simulink model "sysmod1"  (R2019a)
settings: Solver=ode23t  StartTime=0.0  StopTime=2  MaxStep=1e-6  MinStep=1e-7  RelTol=1e-3  EnableMultiTasking=on
values from neighbouring files (symbols this model uses):
  AedivR = pi*hp    (= 0.141371669412)    [setpara1.m]
  Dign = 1    [setpara1.m]
  Dm = 19    [setpara1.m]
  E_const = volpersec / E_spark    (= 5.35724220928e-09)    [setpara1.m]
  init_ediff = 50e-6    (= 5e-05)    [setpara1.m]
  Iref = 5    [setpara1.m]
  mm_dis = 100e-6    (= 0.0001)    [setpara1.m]
  Rsp = 1    [setpara1.m]
  SV = 35    [setpara1.m]
  SVoffset = 2    [setpara1.m]
  Td = Tign + Tm    (= 0.0002)    [setpara1.m]
  Tign = Dign / 100 * Tmach    (= 1e-05)    [setpara1.m]
  Tmach = 1/fmach    (= 0.001)    [setpara1.m]
  Vref = 70    [setpara1.m]
  w1 = 2*pi*f1    (= 62.8318530718)    [setpara1.m]
  wireRad = 90e-6    (= 9e-05)    [setpara1.m]
  wo = 2*pi*fo    (= 62.8318530718)    [setpara1.m]
libraries: powerlib x11, simulink x4
settings Model: Creator=FC Lab  LastModifiedBy=Prakhar
settings SolverCC: AlgebraicLoopSolver=LineSearch
settings DataIOCC: LimitDataPoints=on  ReturnWorkspaceOutputs=off
settings OptimizationCC: LifeSpan=inf
settings DebuggingCC: AllowSymbolicDim=off  SFUnexpectedBacktrackingDiag=warning  SFNoUnconditionalDefaultTransitionDiag=warning  SFExecutionAtInitializationDiag=none  ArithmeticOperatorsInVariantConditions=warning
settings ModelReferenceCC: PropagateSignalLabelsOutOfModel=off
settings SFSimCC: SimUseLocalCustomCode=off
settings RTWCC: RTWUseLocalCustomCode=off
settings CodeAppCC: StateflowObjectComments=on
settings GRTTargetCC: TargetLangStandard=C89/C90 (ANSI)
settings ConfigComp: CovMetricSettings=dw  CovHtmlReporting=on  CovSaveCumulativeToWorkspaceVar=on  CovSaveSingleToWorkspaceVar=on  CovExternalEMLEnable=off
settings SimscapeCC: SimscapeNormalizeSystem=off

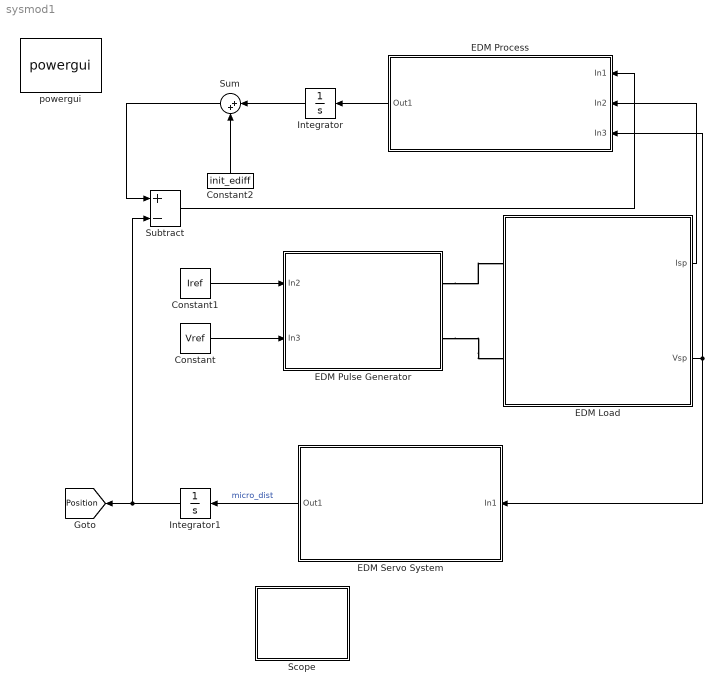
== system sysmod1 ==
  Constant : Constant  Value=Vref
  Constant1 : Constant  Value=Iref
  Constant2 : Constant  Value=init_ediff
  "EDM Load " : Subsystem
  EDM Process : Subsystem
  "EDM Pulse Generator " : Subsystem
  EDM Servo System : Subsystem
  Integrator : Integrator
  Integrator1 : Integrator
  "Scope " : Subsystem
  Subtract : Sum  Inputs=+-
  Sum : Sum  Inputs=|++
  powergui : powerlib/powergui  Priority=1  SimulationMode=Continuous  SampleTime=5e-07  frequency=60  Iterations=50  frequencyindice=0  Pbase=100e6  ErrMax=1e-4  UnitsV=kV  UnitsW=MW  buscounter=0  FunctionMessages=off  echomessages=off  EnableUseOfTLC=off  CurrentSourceSwitches=off  DisableSnubberDevices=off  DisableRonSwitches=off  DisableVfSwitches=off  DisplayEquations=off  AutomaticDiscreteSolvers=off  SolverType=Backward Euler  Interpol=off  ExternalGateDelay=off  methode=off  Ts=0  x0status=zero  SPID=on  SwTol=0  HookPort=off  NonlinearTolerance=0  nMaxIteration=15  ContinueOnMaxIteration=off  RestoreLinks=warning  ResistiveCurrentMeasurement=off  Frange=[0:2:500]  Ylog=off  Xlog=on  ShowGrid=off  save=off  variable=ZData  structure=ScopeData  ZoomFFT=off  StartTime=0.0  cycles=5  DisplayStyle=2  fundamental=50  FreqAxis=off  MaxFrequency=50000  frequencyindicesteady=1  RmsSteady=1  display=off
      settings: SourceProductName=Simscape Electrical
  tag scope: Position=global
  wires:
  Constant1/1 -> "EDM Pulse Generator "/1(In2)
  Constant/1 -> "EDM Pulse Generator "/2(In3)
  "EDM Load "/2(Vsp) -> EDM Servo System/1(In1), EDM Process/3(In3)
  EDM Process/1(Out1) -> Integrator/1
  EDM Servo System/1(Out1) -> Integrator1/1  "micro_dist"
  Integrator1/1 -> Subtract/2, [Position]
  Constant2/1 -> Sum/2
  Integrator/1 -> Sum/1
  Sum/1 -> Subtract/1
  Subtract/1 -> EDM Process/1(In1)
  "EDM Load "/1(Isp) -> EDM Process/2(In2)
  connections:
  "EDM Pulse Generator "/RConn1 -- "EDM Load "/LConn1
  "EDM Pulse Generator "/RConn2 -- "EDM Load "/LConn2

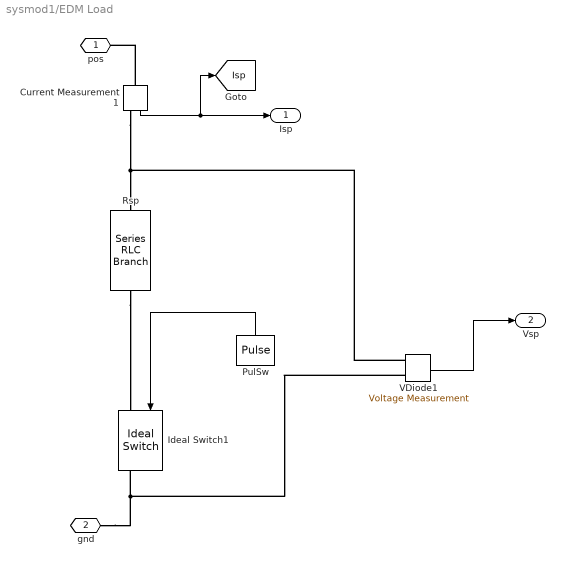
== system sysmod1/EDM Load  ==
  Current Measurement1 : powerlib/Measurements/Current Measurement  PhasorSimulation=off  OutputType=Complex  PSBequivalent=0
      settings: SourceProductName=Simscape Electrical
  Ideal Switch1 : powerlib/Power Electronics/Ideal Switch  Ron=0.001  Lon=0  IC=0  Rs=1e5  Cs=inf  Measurements=on
      settings: SourceProductName=Simscape Electrical
  PulSw : DiscretePulseGenerator  PulseType=Time based  Period=Tmach  PulseWidth=Dm  PhaseDelay=Tign
  Rsp : powerlib/Elements/Series RLC Branch  LConnTagsString=__new0  RConnTagsString=__new0  BranchType=R  Resistance=Rsp  Inductance=3e-6  SetiL0=off  InitialCurrent=0  Capacitance=1e-6  Setx0=off  InitialVoltage=0  Measurements=None
      settings: SourceProductName=Simscape Electrical
  VDiode1 : powerlib/Measurements/Voltage Measurement  PhasorSimulation=off  OutputType=Complex  PSBequivalent=0
      settings: SourceProductName=Simscape Electrical
  pos : PMIOPort  Side=Left
  gnd : PMIOPort  Port=2  Side=Left
  Isp : Outport
  Vsp : Outport  Port=2
  tag scope: Isp=global
  wires:
  PulSw/1 -> Ideal Switch1/1
  Current Measurement1/1 -> [Isp], Isp/1
  VDiode1/1 -> Vsp/1
  connections:
  gnd/RConn1 -- VDiode1/LConn2 -- Ideal Switch1/RConn1
  Current Measurement1/LConn1 -- pos/RConn1
  Current Measurement1/RConn1 -- VDiode1/LConn1 -- Rsp/LConn1
  Rsp/RConn1 -- Ideal Switch1/LConn1

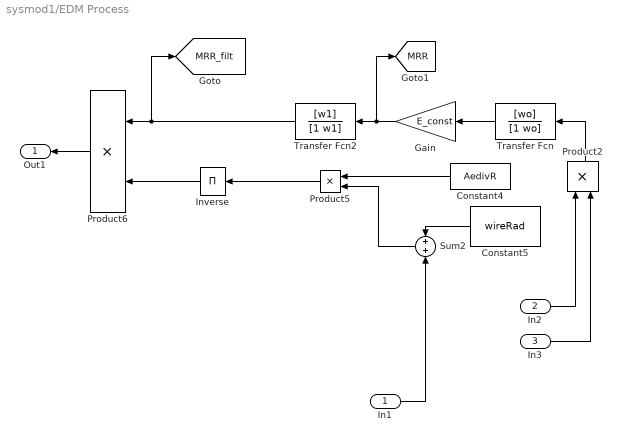
== system sysmod1/EDM Process ==
  In1 : Inport
  In2 : Inport  Port=2
  In3 : Inport  Port=3
  Constant4 : Constant  Value=AedivR
  Constant5 : Constant  Value=wireRad
  Gain : Gain  Gain=E_const
  "Inverse " : Product  Inputs=1
  Product2 : Product
  Product5 : Product
  Product6 : Product
  Sum2 : Sum
  Transfer Fcn : TransferFcn  Numerator=[wo]  Denominator=[1 wo]
  Transfer Fcn2 : TransferFcn  Numerator=[w1]  Denominator=[1 w1]
  Out1 : Outport
  tag scope: MRR=global, MRR_filt=global
  wires:
  Sum2/1 -> Product5/2
  Product6/1 -> Out1/1
  Constant4/1 -> Product5/1
  Product2/1 -> Transfer Fcn/1
  Constant5/1 -> Sum2/1
  "Inverse "/1 -> Product6/2
  Transfer Fcn/1 -> Gain/1
  Product5/1 -> "Inverse "/1
  Transfer Fcn2/1 -> [MRR_filt], Product6/1
  Gain/1 -> [MRR], Transfer Fcn2/1
  In1/1 -> Sum2/2
  In2/1 -> Product2/1
  In3/1 -> Product2/2

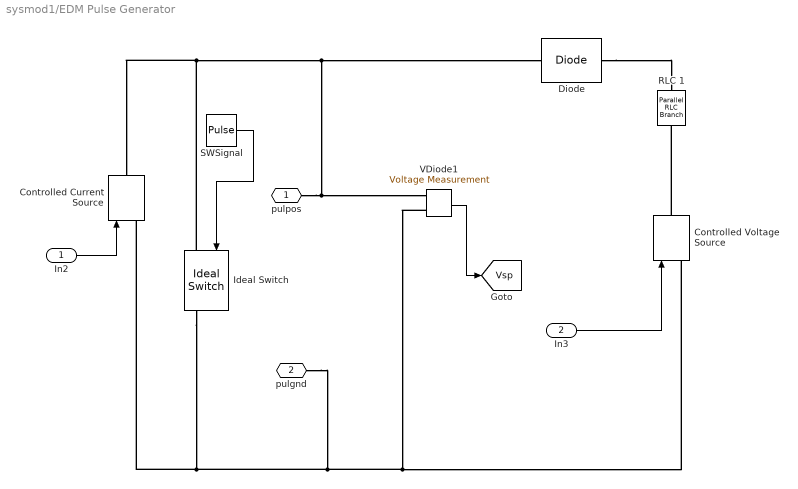
== system sysmod1/EDM Pulse Generator  ==
  In2 : Inport
  In3 : Inport  Port=2
  " RLC 1" : powerlib/Elements/Parallel RLC Branch  LConnTagsString=a  RConnTagsString=__new0  BranchType=R  Resistance=0.001  Inductance=1e-3  SetiL0=off  InitialCurrent=0  Capacitance=0.3e-6  Setx0=off  InitialVoltage=0  Measurements=None
      settings: SourceProductName=Simscape Electrical
  Controlled Current Source : powerlib/Electrical Sources/Controlled Current Source  Initialize=on  Source_Type=AC  Amplitude=0  Phase=0  Frequency=0  Measurements=None
      settings: SourceProductName=Simscape Electrical
  Controlled Voltage Source : powerlib/Electrical Sources/Controlled Voltage Source  Initialize=on  Source_Type=AC  Amplitude=0  Phase=0  Frequency=0  Measurements=None
      settings: SourceProductName=Simscape Electrical
  Diode : powerlib/Power Electronics/Diode  Ron=0.001  Lon=0  Vf=0.8  IC=0  UseSnubber=off  Rs=500  Cs=250e-9  Measurements=off
      settings: SourceProductName=Simscape Electrical
  Ideal Switch : powerlib/Power Electronics/Ideal Switch  Ron=0.001  Lon=0  IC=0  Rs=1e5  Cs=inf  Measurements=on
      settings: SourceProductName=Simscape Electrical
  "SWSignal " : DiscretePulseGenerator  PulseType=Time based  Period=Tmach  PulseWidth=100-(Dm+Dign)  PhaseDelay=Td
  VDiode1 : powerlib/Measurements/Voltage Measurement  PhasorSimulation=off  OutputType=Complex  PSBequivalent=0
      settings: SourceProductName=Simscape Electrical
  pulpos : PMIOPort  Side=Right
  pulgnd : PMIOPort  Port=2  Side=Right
  tag scope: Vsp=global
  wires:
  "SWSignal "/1 -> Ideal Switch/1
  In3/1 -> Controlled Voltage Source/1
  In2/1 -> Controlled Current Source/1
  VDiode1/1 -> [Vsp]
  connections:
  Controlled Voltage Source/RConn1 -- " RLC 1"/RConn1
  VDiode1/LConn2 -- Controlled Voltage Source/LConn1 -- pulgnd/RConn1 -- Controlled Current Source/LConn1 -- Ideal Switch/RConn1
  Diode/RConn1 -- " RLC 1"/LConn1
  Ideal Switch/LConn1 -- VDiode1/LConn1 -- pulpos/RConn1 -- Diode/LConn1 -- Controlled Current Source/RConn1

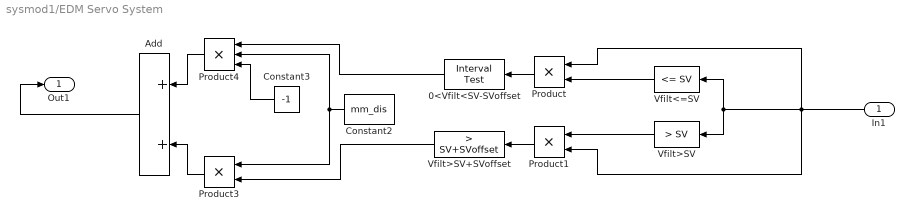
== system sysmod1/EDM Servo System ==
  In1 : Inport
  0<Vfilt<SV-SVoffset : simulink/Logic and Bit Operations/Interval Test  IntervalClosedRight=off  uplimit=SV-SVoffset  IntervalClosedLeft=off  lowlimit=0  OutDataTypeStr=boolean
  Add : Sum
  Constant2 : Constant  Value=mm_dis
  Constant3 : Constant  Value=-1
  Product : Product
  Product1 : Product
  Product3 : Product
  Product4 : Product  Inputs=3
  "Vfilt<=SV " : simulink/Logic and Bit Operations/Compare To Constant  relop=<=  const=SV  OutDataTypeStr=boolean
  "Vfilt>SV " : simulink/Logic and Bit Operations/Compare To Constant  relop=>  const=SV  OutDataTypeStr=boolean
  "Vfilt>SV+SVoffset " : simulink/Logic and Bit Operations/Compare To Constant  relop=>  const=SV+SVoffset  OutDataTypeStr=boolean
  Out1 : Outport
  wires:
  In1/1 -> "Vfilt>SV "/1, "Vfilt<=SV "/1, Product/1, Product1/2
  "Vfilt<=SV "/1 -> Product/2
  Product3/1 -> Add/2
  Constant3/1 -> Product4/3
  Product4/1 -> Add/1
  "Vfilt>SV "/1 -> Product1/1
  Product/1 -> 0<Vfilt<SV-SVoffset/1
  Constant2/1 -> Product4/2, Product3/1
  0<Vfilt<SV-SVoffset/1 -> Product4/1
  Product1/1 -> "Vfilt>SV+SVoffset "/1
  "Vfilt>SV+SVoffset "/1 -> Product3/2
  Add/1 -> Out1/1

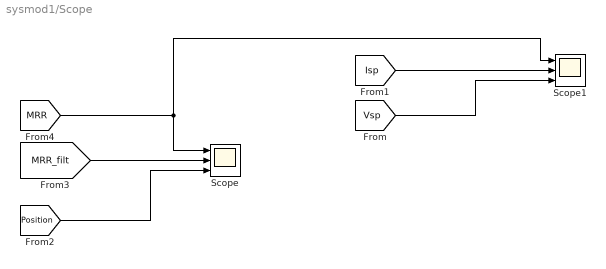
== system sysmod1/Scope  ==
  Scope : Scope  NumInputPorts=3
  Scope1 : Scope  NumInputPorts=3
  wires:
  [MRR_filt] -> Scope/2
  [Isp] -> Scope1/2
  [Vsp] -> Scope1/3
  [MRR] -> Scope/1, Scope1/1
  [Position] -> Scope/3
